simulink model "AB2L3v2015a"  (R2015a)
settings: Solver=ode45  SolverMode=SingleTasking  StartTime=0.0  StopTime=10*pi  FixedStep=.01*pi  RelTol=1e-3
libraries: cstblocks x2
settings Model: CovMetricSettings=dwe  CovHtmlReporting=off  covSaveCumulativeToWorkspaceVar=off  CovSaveSingleToWorkspaceVar=off  CovExternalEMLEnable=on  Creator=root  LastModifiedBy=root
settings DataIOCC: LimitDataPoints=off  SaveFormat=Dataset
settings DebuggingCC: SFUnexpectedBacktrackingDiag=error  SFNoUnconditionalDefaultTransitionDiag=error
settings HardwareCC: ProdBitPerPointer=64  ProdLargestAtomicFloat=Float  ProdIntDivRoundTo=Zero  ProdEndianess=LittleEndian  ProdHWDeviceType=Specified
settings ModelReferenceCC: PropagateSignalLabelsOutOfModel=on
settings SFSimCC: SimUseLocalCustomCode=on
settings RTWCC: RTWUseLocalCustomCode=on
settings GRTTargetCC: TargetLangStandard=C99 (ISO)  GeneratePreprocessorConditionals=Use local settings

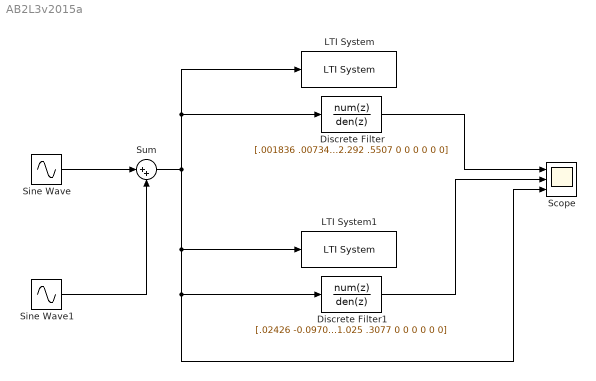
== system AB2L3v2015a ==
  Discrete Filter : DiscreteFilter  Numerator=[.001836 .007344 .01102 .007344 .001836 0 0 0 0 0 0]  Denominator=[1 -3.054 3.829 -2.292 .5507 0 0 0 0 0 0]
  Discrete Filter1 : DiscreteFilter  Numerator=[.02426 -0.09704 0.1456 -.09704 .02426 0 0 0 0 0 0]  Denominator=[1 1.608 1.757 1.025 .3077 0 0 0 0 0 0]
  LTI System : cstblocks/LTI System  sys=H_lp  IC=[]
  LTI System1 : cstblocks/LTI System  sys=H_z  IC=[]
  Scope : Scope  NumInputPorts=3
      settings: TimeRange=auto  ShowLegends=on  MaxDataPoints=5000  SaveToWorkspace=off  SaveName=ScopeData  YMin=-2.48548~-5~-5  YMax=2.43414~5~5  SampleTime=-1
  Sine Wave : Sin  Frequency=2*pi*.1  SampleTime=0
  Sine Wave1 : Sin  Frequency=2*pi*.9  SampleTime=0
  Sum : Sum  Inputs=|++
  wires:
  Sine Wave/1 -> Sum/1
  Sine Wave1/1 -> Sum/2
  Discrete Filter1/1 -> Scope/2
  Discrete Filter/1 -> Scope/1
  Sum/1 -> Discrete Filter1/1, Scope/3, LTI System1/1, LTI System/1, Discrete Filter/1
